simulink model "sampleModel1657"  (R2023a)
settings: Solver=VariableStepAuto  StartTime=0.0  StopTime=10.0  RelTol=1e-3
libraries: hdlsllib x3
settings Model: Creator=user1  LastModifiedBy=user1

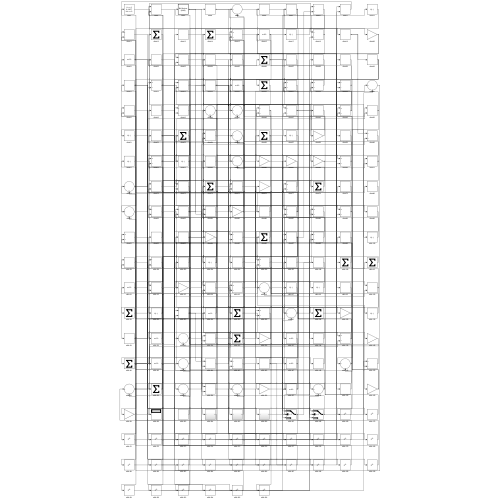
[thumbnail: Simulink's stored preview of the top-level diagram]
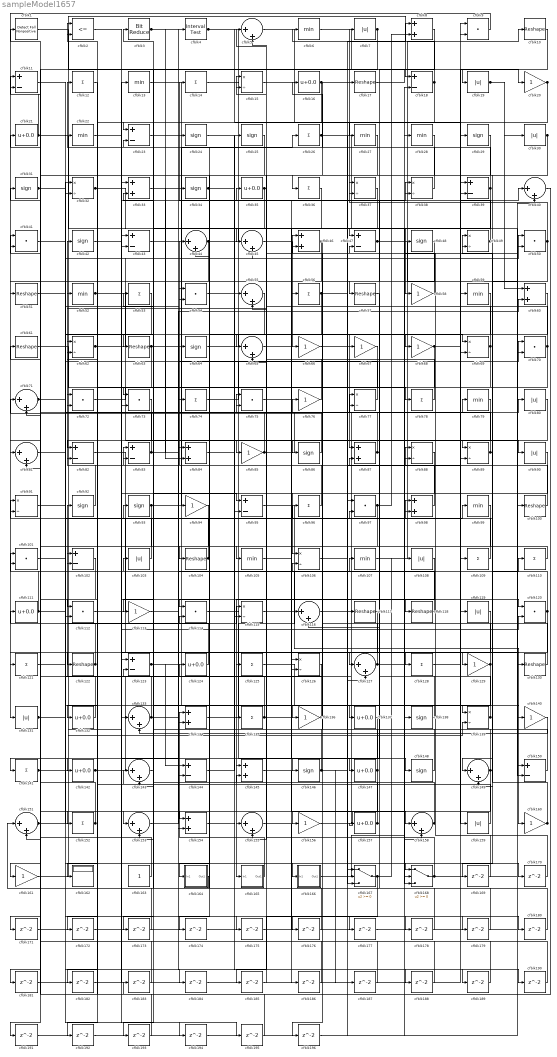
== system sampleModel1657 ==
  cfblk1 : hdlsllib/Logic and Bit Operations/Detect Fall Nonpositive  vinit=0  OutDataTypeStr=boolean
  cfblk{10,17,51,57,61,63,100,104,117..118,122,130} (12 alike) : Reshape
  cfblk{9,41,50,54,70,72..73,75,97,101,112,114,120} (13 alike) : DotProduct  OutDataTypeStr=Inherit: Inherit via internal rule
  cfblk{11,18,23,39,43,47,82..83,95,102,123,144,150} (13 alike) : Sum  Inputs=+-
  cfblk{7,19,30,80,90,103,108,119,131,159} (10 alike) : Abs  SaturateOnIntegerOverflow=off
  cfblk{6,13,22,27..28,52,59,79,99,105,107} (11 alike) : MinMax
  cfblk{15,32,37..38,49,62,69,77,88..89,91,106,115,126,139} (15 alike) : Product  Inputs=*/  RndMeth=Zero  SaturateOnIntegerOverflow=on
  cfblk{12,14,26,36,53,56,74,78,96,109..110,121,125,128,135,141,152} (17 alike) : Sum  Inputs=+
  cfblk{16,21,35,111,124,132,137,142,147,157} (10 alike) : Bias  Bias=0.0  SaturateOnIntegerOverflow=off
  cfblk{20,58,66..68,76,85,94,113,129,136,140,156,160..161} (15 alike) : Gain
  cfblk{5,40,44..45,55,65,71,81,116,127,133,143,149,151,153,155,158} (17 alike) : Sum  Inputs=|++
  cfblk{8,33,46,60,84,87,98,134,145,154} (10 alike) : Sum
  cfblk{24..25,29,31,34,42,48,64,86,92..93,138,146,148} (14 alike) : Signum
  cfblk162 : Display
  cfblk163 : Constant  SampleTime=-1
  cfblk164 : Subsystem
      settings: LibrarySourceBlock=|
      | hdlsllib/Ports &
      | Subsystems/Subsystem
  cfblk165 : Subsystem
      settings: LibrarySourceBlock=|
      | hdlsllib/Ports &
      | Subsystems/Subsystem
  cfblk166 : Subsystem
      settings: LibrarySourceBlock=|
      | hdlsllib/Ports &
      | Subsystems/Subsystem
  cfblk167 : Switch  SaturateOnIntegerOverflow=off  InputSameDT=off
  cfblk168 : Switch  SaturateOnIntegerOverflow=off  InputSameDT=off
  cfblk{169..196} (28 alike) : Delay  SampleTime=1
  cfblk2 : RelationalOperator  Operator=<=  OutDataTypeStr=boolean  InputSameDT=off
  cfblk3 : hdlsllib/Logic and Bit Operations/Bit Reduce  mode=AND
  cfblk4 : hdlsllib/Logic and Bit Operations/Interval Test  IntervalClosedRight=on  uplimit=0.5  IntervalClosedLeft=on  lowlimit=-0.5  OutDataTypeStr=boolean
  wires:
  cfblk4/1 -> cfblk128/1, cfblk27/1
  cfblk107/1 -> cfblk10/1
  cfblk141/1 -> cfblk18/1, cfblk139/2, cfblk120/2, cfblk194/1
  cfblk95/1 -> cfblk160/1
  cfblk90/1 -> cfblk106/1
  cfblk44/1 -> cfblk47/1, cfblk153/2
  cfblk150/1 -> cfblk76/1
  cfblk133/1 -> cfblk92/1, cfblk77/2
  cfblk165/1(Out1) -> cfblk134/1
  cfblk38/1 -> cfblk12/1
  cfblk108/1 -> cfblk165/1(In1)
  cfblk82/1 -> cfblk129/1
  cfblk120/1 -> cfblk134/2, cfblk49/1
  cfblk6/1 -> cfblk19/1
  cfblk156/1 -> cfblk79/1
  cfblk23/1 -> cfblk136/1
  cfblk147/1 -> cfblk103/1, cfblk181/1
  cfblk64/1 -> cfblk69/1
  cfblk158/1 -> cfblk157/1, cfblk23/2
  cfblk72/1 -> cfblk78/1
  cfblk161/1 -> cfblk115/1
  cfblk60/1 -> cfblk154/1
  cfblk59/1 -> cfblk87/1
  cfblk43/1 -> cfblk130/1
  cfblk92/1 -> cfblk42/1
  cfblk146/1 -> cfblk88/1, cfblk114/2, cfblk187/1
  cfblk9/1 -> cfblk131/1
  cfblk93/1 -> cfblk26/1, cfblk60/2, cfblk191/1
  cfblk7/1 -> cfblk161/1, cfblk23/1
  cfblk63/1 -> cfblk122/1, cfblk95/2
  cfblk19/1 -> cfblk60/1, cfblk30/1
  cfblk142/1 -> cfblk69/2, cfblk37/2
  cfblk153/1 -> cfblk94/1
  cfblk151/1 -> cfblk13/1, cfblk124/1
  cfblk98/1 -> cfblk44/1
  cfblk99/1 -> cfblk152/1
  cfblk32/1 -> cfblk138/1, cfblk120/1
  cfblk124/1 -> cfblk102/1
  cfblk166/1(Out1) -> cfblk28/1
  cfblk46/1 -> cfblk156/1, cfblk81/1
  cfblk105/1 -> cfblk99/1
  cfblk29/1 -> cfblk155/1
  cfblk22/1 -> cfblk133/1
  cfblk125/1 -> cfblk140/1
  cfblk100/1 -> cfblk33/2
  cfblk15/1 -> cfblk119/1
  cfblk129/1 -> cfblk101/1, cfblk153/1
  cfblk123/1 -> cfblk145/1, cfblk144/1
  cfblk45/1 -> cfblk66/1
  cfblk109/1 -> cfblk98/1
  cfblk13/1 -> cfblk45/1
  cfblk41/1 -> cfblk166/1(In1)
  cfblk85/1 -> cfblk77/1, cfblk53/1
  cfblk143/1 -> cfblk83/1
  cfblk1/1 -> cfblk59/1
  cfblk149/1 -> cfblk72/1, cfblk49/2, cfblk193/1
  cfblk56/1 -> cfblk155/2, cfblk118/1
  cfblk104/1 -> cfblk3/1, cfblk41/2
  cfblk52/1 -> cfblk89/1, cfblk144/2, cfblk195/1
  cfblk35/1 -> cfblk104/1, cfblk65/2
  cfblk20/1 -> cfblk82/1, cfblk73/1
  cfblk55/1 -> cfblk164/1(In1)
  cfblk148/1 -> cfblk93/1
  cfblk110/1 -> cfblk105/1
  cfblk25/1 -> cfblk114/1
  cfblk73/1 -> cfblk112/1
  cfblk139/1 -> cfblk74/1, cfblk116/2
  cfblk76/1 -> cfblk52/1
  cfblk18/1 -> cfblk43/2, cfblk6/1
  cfblk34/1 -> cfblk68/1, cfblk179/1, cfblk180/1
  cfblk69/1 -> cfblk15/1, cfblk88/2
  cfblk127/1 -> cfblk46/1, cfblk50/1
  cfblk121/1 -> cfblk54/1
  cfblk57/1 -> cfblk137/1
  cfblk102/1 -> cfblk141/1
  cfblk91/1 -> cfblk168/1
  cfblk8/1 -> cfblk57/1
  cfblk21/1 -> cfblk159/1, cfblk139/1, cfblk11/2
  cfblk80/1 -> cfblk154/2
  cfblk78/1 -> cfblk54/2
  cfblk77/1 -> cfblk64/1
  cfblk119/1 -> cfblk168/2
  cfblk167/1 -> cfblk108/1, cfblk185/1
  cfblk112/1 -> cfblk56/1
  cfblk71/1 -> cfblk32/1, cfblk50/2
  cfblk96/1 -> cfblk22/1
  cfblk152/1 -> cfblk31/1, cfblk91/1
  cfblk50/1 -> cfblk7/1, cfblk149/2
  cfblk114/1 -> cfblk167/1
  cfblk157/1 -> cfblk107/1, cfblk15/2
  cfblk106/1 -> cfblk8/1
  cfblk111/1 -> cfblk101/2, cfblk190/1
  cfblk160/1 -> cfblk96/1, cfblk91/2
  cfblk2/1 -> cfblk127/1
  cfblk26/1 -> cfblk58/1, cfblk168/3
  cfblk17/1 -> cfblk20/1
  cfblk14/1 -> cfblk100/1
  cfblk132/1 -> cfblk21/1
  cfblk88/1 -> cfblk113/1
  cfblk116/1 -> cfblk117/1
  cfblk130/1 -> cfblk71/1
  cfblk144/1 -> cfblk25/1
  cfblk134/1 -> cfblk67/1
  cfblk118/1 -> cfblk62/1
  cfblk3/1 -> cfblk4/1, cfblk84/2, cfblk189/1
  cfblk126/1 -> cfblk123/2
  cfblk11/1 -> cfblk65/1
  cfblk53/1 -> cfblk112/2
  cfblk113/1 -> cfblk110/1
  cfblk68/1 -> cfblk147/1, cfblk40/1
  cfblk49/1 -> cfblk14/1, cfblk38/2
  cfblk94/1 -> cfblk132/1
  cfblk33/1 -> cfblk126/2
  cfblk5/1 -> cfblk109/1
  cfblk83/1 -> cfblk34/1, cfblk11/1, cfblk178/1
  cfblk159/1 -> cfblk72/2
  cfblk24/1 -> cfblk55/1
  cfblk37/1 -> cfblk85/1
  cfblk39/1 -> cfblk16/1, cfblk173/1
  cfblk65/1 -> cfblk90/1
  cfblk31/1 -> cfblk167/2, cfblk184/1
  cfblk97/1 -> cfblk125/1, cfblk142/1, cfblk167/3, cfblk48/1
  cfblk61/1 -> cfblk116/1
  cfblk74/1 -> cfblk9/2
  cfblk168/1 -> cfblk143/1, cfblk40/2
  cfblk16/1 -> cfblk36/1, cfblk17/1, cfblk143/2
  cfblk103/1 -> cfblk61/1
  cfblk51/1 -> cfblk32/2
  cfblk163/1 -> cfblk71/2
  cfblk62/1 -> cfblk45/2, cfblk95/1
  cfblk135/1 -> cfblk41/1, cfblk38/1, cfblk84/1
  cfblk48/1 -> cfblk146/1
  cfblk128/1 -> cfblk29/1
  cfblk47/1 -> cfblk150/2, cfblk8/2
  cfblk75/1 -> cfblk148/1
  cfblk86/1 -> cfblk62/2
  cfblk28/1 -> cfblk63/1
  cfblk30/1 -> cfblk51/1, cfblk149/1, cfblk73/2
  cfblk79/1 -> cfblk162/1
  cfblk138/1 -> cfblk106/2
  cfblk164/1(Out1) -> cfblk151/1
  cfblk136/1 -> cfblk135/1, cfblk75/2
  cfblk70/1 -> cfblk5/2, cfblk196/1
  cfblk131/1 -> cfblk97/2, cfblk75/1
  cfblk89/1 -> cfblk24/1, cfblk169/1
  cfblk81/1 -> cfblk70/1
  cfblk122/1 -> cfblk121/1, cfblk111/1
  cfblk10/1 -> cfblk39/2
  cfblk58/1 -> cfblk35/1
  cfblk140/1 -> cfblk133/2
  cfblk87/1 -> cfblk2/1, cfblk37/1
  cfblk84/1 -> cfblk86/1
  cfblk115/1 -> cfblk80/1
  cfblk27/1 -> cfblk115/2
  cfblk145/1 -> cfblk158/1
  cfblk169/1 -> cfblk46/2
  cfblk66/1 -> cfblk170/1
  cfblk170/1 -> cfblk87/2
  cfblk137/1 -> cfblk171/1
  cfblk171/1 -> cfblk98/2
  cfblk67/1 -> cfblk172/1
  cfblk172/1 -> cfblk150/1
  cfblk173/1 -> cfblk1/1
  cfblk36/1 -> cfblk174/1
  cfblk174/1 -> cfblk89/2
  cfblk101/1 -> cfblk175/1
  cfblk175/1 -> cfblk126/1
  cfblk54/1 -> cfblk176/1
  cfblk176/1 -> cfblk55/2
  cfblk42/1 -> cfblk177/1
  cfblk177/1 -> cfblk9/1
  cfblk178/1 -> cfblk44/2
  cfblk179/1 -> cfblk47/2
  cfblk180/1 -> cfblk83/2
  cfblk181/1 -> cfblk43/1
  cfblk117/1 -> cfblk182/1
  cfblk182/1 -> cfblk39/1
  cfblk40/1 -> cfblk183/1
  cfblk183/1 -> cfblk102/2
  cfblk184/1 -> cfblk97/1
  cfblk185/1 -> cfblk5/1
  cfblk155/1 -> cfblk186/1
  cfblk186/1 -> cfblk33/1
  cfblk187/1 -> cfblk123/1
  cfblk154/1 -> cfblk188/1
  cfblk188/1 -> cfblk145/2
  cfblk189/1 -> cfblk151/2
  cfblk190/1 -> cfblk82/2
  cfblk191/1 -> cfblk158/2
  cfblk12/1 -> cfblk192/1
  cfblk192/1 -> cfblk18/2
  cfblk193/1 -> cfblk81/2
  cfblk194/1 -> cfblk70/2
  cfblk195/1 -> cfblk2/2
  cfblk196/1 -> cfblk127/2

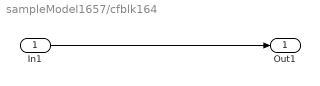
== system sampleModel1657/cfblk164 ==
  In1 : Inport
  Out1 : Outport
  wires:
  In1/1 -> Out1/1

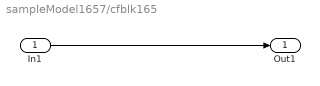
== system sampleModel1657/cfblk165 ==
  In1 : Inport
  Out1 : Outport
  wires:
  In1/1 -> Out1/1

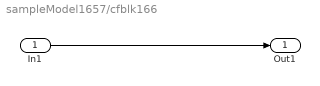
== system sampleModel1657/cfblk166 ==
  In1 : Inport
  Out1 : Outport
  wires:
  In1/1 -> Out1/1
